simulink model "advisor_ess_options"  (Simulink 2.20)
settings: Solver=ode1  StartTime=0.0  StopTime=500  FixedStep=1  RelTol=1e-3
values from neighbouring files (symbols this model uses):
  amb_tmp = vinf.test.ambtmp    [RW_execute.m]
  cyc_mph = [time speed]    [DataCompareFigControl.m]    (also in J17_FUDS.m = [time_vec speed_vec]; J17_HFEDS.m = [time_vec speed_vec]; J17_SC03.m = [time_vec speed_vec]; J17_UDDS.m = [time_vec speed_vec])
  ess_init_soc = vinf.test.ess_init_soc.FUDS    [J17_FUDS.m]    (also in J17_HFEDS.m = vinf.test.ess_init_soc.HWFET; J17_SC03.m = vinf.test.ess_init_soc.SC03; J17_UDDS.m = vinf.test.ess_init_soc.UDDS; J17_US06.m = vinf.test.ess_init_soc.US06)
undefined symbols (not defined in the file or in its folder): air_cp, enable_stop, ess_coulombic_eff, ess_max_ah_cap, ess_max_p, ess_max_p_soc, ess_max_volts, ess_min_volts, ess_MMi, ess_MMo, ess_mod_airflow, ess_mod_cp, ess_mod_init_tmp, ess_module_mass, ess_module_num, ess_on, ess_set_tmp, ess_th_calc, ess_th_res_off, ess_th_res_on, ess_tmp, fund_byu, fund_byuop, mc_min_volts, t_soc
(part 2 of 2)

== system advisor_ess_options/energy storage <ess> nnet/NNet/Neural Network/Layer 2/LW{2,1} ==
  "ad{2,1}" : Inport  Port=1  PortWidth=3  SampleTime=-1
  "IW{2,1}(1,:)'" : Constant  Value=[-0.2776092;-2.6799360000000001;-2.2138360000000001]
      mask Display: disp('weights')
  "IW{2,1}(2,:)'" : Constant  Value=[3.601111;2.064257;0.86618079999999997]
      mask Display: disp('weights')
  Mux : Mux  Inputs=2
  dotprod1 : Subsystem
  dotprod2 : Subsystem
  "lz{2,1}" : Outport  Port=1  InitialOutput=0
  wires:
  "IW{2,1}(1,:)'"/1 -> dotprod1/1(w)
  dotprod1/1(z) -> Mux/1
  "IW{2,1}(2,:)'"/1 -> dotprod2/1(w)
  "ad{2,1}"/1 -> dotprod1/2(p), dotprod2/2(p)
  dotprod2/1(z) -> Mux/2
  Mux/1 -> "lz{2,1}"/1

== system advisor_ess_options/energy storage <ess> nnet/NNet/Neural Network/Layer 2/logsig ==
  n : Inport  Port=1  PortWidth=-1  SampleTime=-1
  Exp : ElementaryMath  Operator=exp
  Gain : Gain  Gain=-1
  Reciprocal : ElementaryMath  Operator=reciprocal
  Sum : Sum  Inputs=++
  one : Constant  Value=1
  a : Outport  Port=1  InitialOutput=0
  wires:
  Reciprocal/1 -> a/1
  Sum/1 -> Reciprocal/1
  one/1 -> Sum/2
  Exp/1 -> Sum/1
  Gain/1 -> Exp/1
  n/1 -> Gain/1

== system advisor_ess_options/energy storage <ess> nnet/NNet/Neural Network/Layer 1/IW{1,1}/dotprod1 ==
  w : Inport  Port=1  PortWidth=-1  SampleTime=-1
  p : Inport  Port=2  PortWidth=-1  SampleTime=-1
  Dot Product : Subsystem  mask(Dot Product){}
      mask help:
      | Inner (dot) product.
      | y=sum(u1.*u2)
      mask init:
      | t=(0:.1:2*pi)';
      | x=cos(t);
      | y=sin(t);
      mask Help: Computes the inner (dot) product of the inputs: sum(u1.*u2).  The inputs are vectors of the same length. Output is a scalar.
      mask Display: plot(0,0,1,1,x*[0.025 0.07]+0.5,y*[0.025 0.07]+0.5)
  z : Outport  Port=1  InitialOutput=0
  wires:
  Dot Product/1(out_1) -> z/1
  p/1 -> Dot Product/2(in_2)
  w/1 -> Dot Product/1(in_1)

== system advisor_ess_options/energy storage <ess> nnet/NNet/Neural Network/Layer 1/IW{1,1}/dotprod2 ==
  w : Inport  Port=1  PortWidth=-1  SampleTime=-1
  p : Inport  Port=2  PortWidth=-1  SampleTime=-1
  Dot Product : Subsystem  mask(Dot Product){}
      mask help:
      | Inner (dot) product.
      | y=sum(u1.*u2)
      mask init:
      | t=(0:.1:2*pi)';
      | x=cos(t);
      | y=sin(t);
      mask Help: Computes the inner (dot) product of the inputs: sum(u1.*u2).  The inputs are vectors of the same length. Output is a scalar.
      mask Display: plot(0,0,1,1,x*[0.025 0.07]+0.5,y*[0.025 0.07]+0.5)
  z : Outport  Port=1  InitialOutput=0
  wires:
  Dot Product/1(out_1) -> z/1
  p/1 -> Dot Product/2(in_2)
  w/1 -> Dot Product/1(in_1)

== system advisor_ess_options/energy storage <ess> nnet/NNet/Neural Network/Layer 1/IW{1,1}/dotprod3 ==
  w : Inport  Port=1  PortWidth=-1  SampleTime=-1
  p : Inport  Port=2  PortWidth=-1  SampleTime=-1
  Dot Product : Subsystem  mask(Dot Product){}
      mask help:
      | Inner (dot) product.
      | y=sum(u1.*u2)
      mask init:
      | t=(0:.1:2*pi)';
      | x=cos(t);
      | y=sin(t);
      mask Help: Computes the inner (dot) product of the inputs: sum(u1.*u2).  The inputs are vectors of the same length. Output is a scalar.
      mask Display: plot(0,0,1,1,x*[0.025 0.07]+0.5,y*[0.025 0.07]+0.5)
  z : Outport  Port=1  InitialOutput=0
  wires:
  Dot Product/1(out_1) -> z/1
  p/1 -> Dot Product/2(in_2)
  w/1 -> Dot Product/1(in_1)

== system advisor_ess_options/energy storage <ess> nnet/NNet/Neural Network/Layer 2/LW{2,1}/dotprod1 ==
  w : Inport  Port=1  PortWidth=-1  SampleTime=-1
  p : Inport  Port=2  PortWidth=-1  SampleTime=-1
  Dot Product : Subsystem  mask(Dot Product){}
      mask help:
      | Inner (dot) product.
      | y=sum(u1.*u2)
      mask init:
      | t=(0:.1:2*pi)';
      | x=cos(t);
      | y=sin(t);
      mask Help: Computes the inner (dot) product of the inputs: sum(u1.*u2).  The inputs are vectors of the same length. Output is a scalar.
      mask Display: plot(0,0,1,1,x*[0.025 0.07]+0.5,y*[0.025 0.07]+0.5)
  z : Outport  Port=1  InitialOutput=0
  wires:
  Dot Product/1(out_1) -> z/1
  p/1 -> Dot Product/2(in_2)
  w/1 -> Dot Product/1(in_1)

== system advisor_ess_options/energy storage <ess> nnet/NNet/Neural Network/Layer 2/LW{2,1}/dotprod2 ==
  w : Inport  Port=1  PortWidth=-1  SampleTime=-1
  p : Inport  Port=2  PortWidth=-1  SampleTime=-1
  Dot Product : Subsystem  mask(Dot Product){}
      mask help:
      | Inner (dot) product.
      | y=sum(u1.*u2)
      mask init:
      | t=(0:.1:2*pi)';
      | x=cos(t);
      | y=sin(t);
      mask Help: Computes the inner (dot) product of the inputs: sum(u1.*u2).  The inputs are vectors of the same length. Output is a scalar.
      mask Display: plot(0,0,1,1,x*[0.025 0.07]+0.5,y*[0.025 0.07]+0.5)
  z : Outport  Port=1  InitialOutput=0
  wires:
  Dot Product/1(out_1) -> z/1
  p/1 -> Dot Product/2(in_2)
  w/1 -> Dot Product/1(in_1)

== system advisor_ess_options/energy storage <ess> nnet/NNet/Neural Network/Layer 1/IW{1,1}/dotprod1/Dot Product ==
  in_1 : Inport  Port=1  PortWidth=-1  SampleTime=-1
  in_2 : Inport  Port=2  PortWidth=-1  SampleTime=-1
  Product : Product  Inputs=2
  Sum : Sum  Inputs=+
  out_1 : Outport  Port=1  InitialOutput=0
  wires:
  Sum/1 -> out_1/1
  Product/1 -> Sum/1
  in_1/1 -> Product/1
  in_2/1 -> Product/2

== system advisor_ess_options/energy storage <ess> nnet/NNet/Neural Network/Layer 1/IW{1,1}/dotprod2/Dot Product ==
  in_1 : Inport  Port=1  PortWidth=-1  SampleTime=-1
  in_2 : Inport  Port=2  PortWidth=-1  SampleTime=-1
  Product : Product  Inputs=2
  Sum : Sum  Inputs=+
  out_1 : Outport  Port=1  InitialOutput=0
  wires:
  Sum/1 -> out_1/1
  Product/1 -> Sum/1
  in_1/1 -> Product/1
  in_2/1 -> Product/2

== system advisor_ess_options/energy storage <ess> nnet/NNet/Neural Network/Layer 1/IW{1,1}/dotprod3/Dot Product ==
  in_1 : Inport  Port=1  PortWidth=-1  SampleTime=-1
  in_2 : Inport  Port=2  PortWidth=-1  SampleTime=-1
  Product : Product  Inputs=2
  Sum : Sum  Inputs=+
  out_1 : Outport  Port=1  InitialOutput=0
  wires:
  Sum/1 -> out_1/1
  Product/1 -> Sum/1
  in_1/1 -> Product/1
  in_2/1 -> Product/2

== system advisor_ess_options/energy storage <ess> nnet/NNet/Neural Network/Layer 2/LW{2,1}/dotprod1/Dot Product ==
  in_1 : Inport  Port=1  PortWidth=-1  SampleTime=-1
  in_2 : Inport  Port=2  PortWidth=-1  SampleTime=-1
  Product : Product  Inputs=2
  Sum : Sum  Inputs=+
  out_1 : Outport  Port=1  InitialOutput=0
  wires:
  Sum/1 -> out_1/1
  Product/1 -> Sum/1
  in_1/1 -> Product/1
  in_2/1 -> Product/2

== system advisor_ess_options/energy storage <ess> nnet/NNet/Neural Network/Layer 2/LW{2,1}/dotprod2/Dot Product ==
  in_1 : Inport  Port=1  PortWidth=-1  SampleTime=-1
  in_2 : Inport  Port=2  PortWidth=-1  SampleTime=-1
  Product : Product  Inputs=2
  Sum : Sum  Inputs=+
  out_1 : Outport  Port=1  InitialOutput=0
  wires:
  Sum/1 -> out_1/1
  Product/1 -> Sum/1
  in_1/1 -> Product/1
  in_2/1 -> Product/2
